simulink model "chap8_2sim"  (Simulink 5.0)
settings: Solver=ode45  SolverMode=SingleTasking  StartTime=0.0  StopTime=80  FixedStep=0.001  RelTol=1e-3
settings Model: LastModifiedBy=Administrator  ExtModeTrigMode=oneshot  ExtModeArmWhenConnect=off  LimitDataPoints=off  BooleanDataType=off

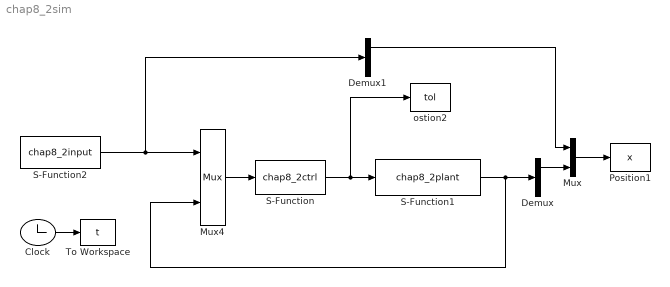
== system chap8_2sim ==
  Clock : Clock
  Demux : Demux  Outputs=2
  Demux1 : Demux  Outputs=2
  Mux : Mux  Inputs=2
  Mux4 : Mux  Inputs=2
  Position1 : ToWorkspace  VariableName=x  SampleTime=-1  SaveFormat=Array
  S-Function : S-Function  FunctionName=chap8_2ctrl
  S-Function1 : S-Function  FunctionName=chap8_2plant
  S-Function2 : S-Function  FunctionName=chap8_2input
  To Workspace : ToWorkspace  VariableName=t  SampleTime=-1  SaveFormat=Array
  ostion2 : ToWorkspace  VariableName=tol  SampleTime=-1  SaveFormat=Array
  wires:
  Mux4/1 -> S-Function/1
  Clock/1 -> To Workspace/1
  S-Function2/1 -> Mux4/1, Demux1/1
  S-Function/1 -> S-Function1/1, ostion2/1
  Mux/1 -> Position1/1
  S-Function1/1 -> Demux/1, Mux4/2
  Demux/1 -> Mux/2
  Demux1/1 -> Mux/1
